simulink model "Copter_Plane_h2g_4_and_1_20210113"  (R2020b)
settings: Solver=ode1  StartTime=0.0  StopTime=50  FixedStep=dt  RelTol=1e-3
values from neighbouring files (symbols this model uses):
  HD = 180/pi    (= 57.2957795131)    [mode_data.m]
undefined symbols (not defined in the file or in its folder): center_WP, GRAVITY_MSS, gyro_x, gyro_y, gyro_z, J, k_aileron, k_aileronL, k_aileronR, k_elevator, k_flap, k_rudder, Kd, Ku, Ld, Ldx, Ldy, Lu, Lux, Luy, m_kg, Newton, pid_vel_xy_derivative, pid_vel_xy_input, pid_vel_xy_integrator, pitch, POSCONTROL_ACC_Z_D, POSCONTROL_ACC_Z_P, POSCONTROL_VEL_XY_D, POSCONTROL_VEL_XY_P, pwm_max, pwm_min, pwm_out, pwm_tail, Qd, QLd, QLdx, QLdy, QLu, QLux, QLuy, Qu, Raphson, roll, tail_tilt, vel_desired, yaw
libraries: shared6dofsys x3, sharedutil x1, simulink x1, aerolibasang x1
(part 3 of 3)

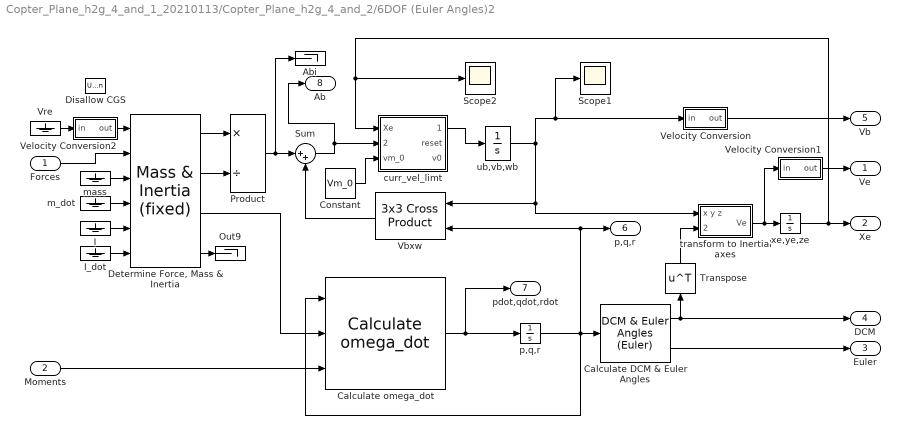
== system Copter_Plane_h2g_4_and_1_20210113/Copter_Plane_h2g_4_and_2/6DOF (Euler Angles)2 ==
  Forces : Inport  Unit=N  PortDimensions=3
  Moments : Inport  Port=2  Unit=N*m  PortDimensions=3
  Abi : Terminator
  Calculate DCM & Euler Angles : shared6dofsys/DCM & Euler Angles (Euler)  aMode=aMode
      settings: SourceProductBaseCode=AE,PW,MT,UV,VE,VP
  Calculate omega_dot : shared6dofsys/Calculate omega_dot  aMode=aMode
      settings: SourceProductBaseCode=AE,PW,MT,UV,VE,VP
  Constant : Constant  Value=Vm_0
  "Determine Force, Mass & Inertia" : shared6dofsys/Mass & Inertia (fixed)  aMode=aMode
      settings: SourceProductBaseCode=AE,PW,MT,UV,VE,VP
  Disallow CGS : UnitConfiguration  UnitSystemsStr=English,SI,SI (extended)  AllowAllUnitSystems=off
  I : Ground
  I_dot : Ground
  Out9 : Terminator
  Product : Product  Inputs=*/  SaturateOnIntegerOverflow=on  OutDataTypeStr=Inherit: Same as first input
  Scope1 : Scope
  Scope2 : Scope
  Sum : Sum  Inputs=|++  SaturateOnIntegerOverflow=on
  Transpose : Math  Operator=transpose  SignedPower=on  SaturateOnIntegerOverflow=on
  Vbxw : sharedutil/3x3 Cross Product  aMode=aMode
      settings: SourceProductBaseCode=AE,PW,MT,UV,VE,VP
  Velocity Conversion : Subsystem
  Velocity Conversion1 : Subsystem
  Velocity Conversion2 : Subsystem
  Vre : Ground
  curr_vel_limt : MATLAB Function  TreatAsAtomicUnit=on
  m_dot : Ground
  mass : Ground
  "p,q,r " : Integrator  InitialCondition=pm_0  ContinuousStateAttributes=pm_statename
  "transform to Inertial axes " : Subsystem  mask(Vector Transformation){}
      mask Display: disp('L_EB')
  ub,vb,wb : Integrator  InitialCondition=Vm_0  UpperSaturationLimit=[inf inf 0]  ContinuousStateAttributes=Vm_statename
  xe,ye,ze : Integrator  InitialCondition=xme_0  ContinuousStateAttributes=xme_statename
  Ve : Outport  Unit=m/s  VectorParamsAs1DForOutWhenUnconnected=off
  Xe : Outport  Port=2  Unit=m  VectorParamsAs1DForOutWhenUnconnected=off
  Euler : Outport  Port=3  Unit=rad  VectorParamsAs1DForOutWhenUnconnected=off
  DCM : Outport  Port=4  Unit=1  VectorParamsAs1DForOutWhenUnconnected=off
  Vb : Outport  Port=5  Unit=m/s  VectorParamsAs1DForOutWhenUnconnected=off
  p,q,r : Outport  Port=6  Unit=rad/s  VectorParamsAs1DForOutWhenUnconnected=off
  pdot,qdot,rdot : Outport  Port=7  Unit=rad/s^2  VectorParamsAs1DForOutWhenUnconnected=off
  Ab : Outport  Port=8  Unit=m/s^2  VectorParamsAs1DForOutWhenUnconnected=off
  wires:
  Velocity Conversion1/1(out) -> Ve/1
  Sum/1 -> Ab/1, curr_vel_limt/2(accel_in)
  ub,vb,wb/1 -> "transform to Inertial axes "/1(x y z), Vbxw/1, Scope1/1, Velocity Conversion/1(in)
  Velocity Conversion/1(out) -> Vb/1
  Velocity Conversion2/1(out) -> "Determine Force, Mass & Inertia"/1
  Vre/1 -> Velocity Conversion2/1(in)
  "Determine Force, Mass & Inertia"/1 -> Product/1
  I_dot/1 -> "Determine Force, Mass & Inertia"/6
  I/1 -> "Determine Force, Mass & Inertia"/5
  Calculate omega_dot/1 -> "p,q,r "/1, pdot,qdot,rdot/1
  "Determine Force, Mass & Inertia"/4 -> Out9/1
  m_dot/1 -> "Determine Force, Mass & Inertia"/4
  "Determine Force, Mass & Inertia"/2 -> Product/2
  mass/1 -> "Determine Force, Mass & Inertia"/3
  Transpose/1 -> "transform to Inertial axes "/2(transform coefficients)
  Calculate DCM & Euler Angles/1 -> Transpose/1, DCM/1
  Product/1 -> Sum/1, Abi/1
  Forces/1 -> "Determine Force, Mass & Inertia"/2
  Moments/1 -> Calculate omega_dot/3
  "p,q,r "/1 -> Calculate DCM & Euler Angles/1, Calculate omega_dot/1, p,q,r/1, Vbxw/2
  "transform to Inertial axes "/1(Ve) -> xe,ye,ze/1, Velocity Conversion1/1(in)
  xe,ye,ze/1 -> Scope2/1, curr_vel_limt/1(Xe), Xe/1
  Vbxw/1 -> Sum/2
  Calculate DCM & Euler Angles/2 -> Euler/1
  "Determine Force, Mass & Inertia"/3 -> Calculate omega_dot/2
  curr_vel_limt/1(accel_o) -> ub,vb,wb/1
  Constant/1 -> curr_vel_limt/3(vm_0)

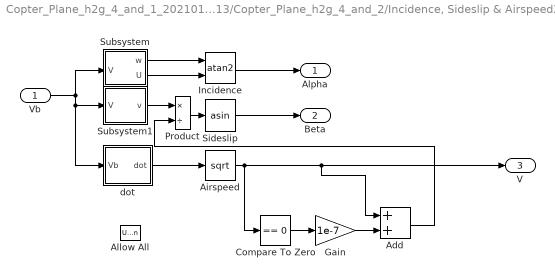
== system Copter_Plane_h2g_4_and_1_20210113/Copter_Plane_h2g_4_and_2/Incidence, Sideslip & Airspeed2 ==
  Vb : Inport
  Add : Sum
  Airspeed : Sqrt  AlgorithmType=Newton-Raphson  SaturateOnIntegerOverflow=on
  Allow All : UnitConfiguration  UnitSystemsStr=English,SI,SI (extended)  AllowAllUnitSystems=off
  Compare To Zero : simulink/Logic and Bit Operations/Compare To Zero  relop===  OutDataTypeStr=boolean
  Gain : Gain  Gain=1e-7
  Incidence : Trigonometry  Operator=atan2
  Product : Product  Inputs=*/  SaturateOnIntegerOverflow=on  OutDataTypeStr=Inherit: Same as first input
  Sideslip : Trigonometry  Operator=asin
  Subsystem : Subsystem
  Subsystem1 : Subsystem
  dot : Subsystem
  Alpha : Outport  Unit=rad  InitialOutput=0  VectorParamsAs1DForOutWhenUnconnected=off
  Beta : Outport  Port=2  Unit=rad  InitialOutput=0  VectorParamsAs1DForOutWhenUnconnected=off
  V : Outport  Port=3  InitialOutput=0  VectorParamsAs1DForOutWhenUnconnected=off
  wires:
  Product/1 -> Sideslip/1
  Subsystem/1(w) -> Incidence/1
  Subsystem/2(U) -> Incidence/2
  dot/1(dot) -> Airspeed/1
  Airspeed/1 -> Compare To Zero/1, Add/1, V/1
  Incidence/1 -> Alpha/1
  Vb/1 -> Subsystem/1(V), Subsystem1/1(V), dot/1(Vb)
  Sideslip/1 -> Beta/1
  Subsystem1/1(v) -> Product/1
  Compare To Zero/1 -> Gain/1
  Gain/1 -> Add/2
  Add/1 -> Product/2

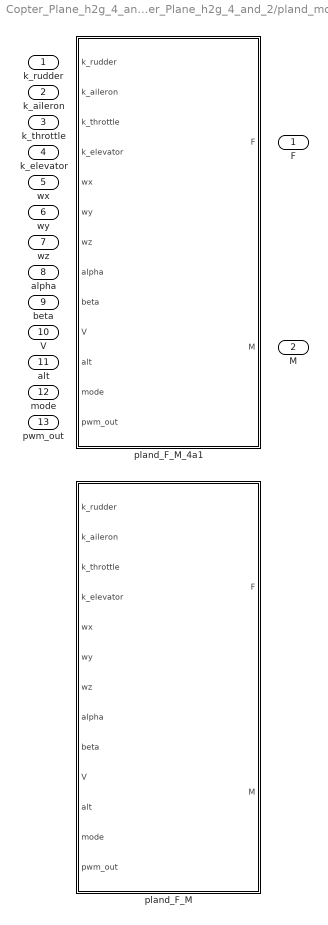
== system Copter_Plane_h2g_4_and_1_20210113/Copter_Plane_h2g_4_and_2/pland_mode ==
  k_rudder : Inport
  k_aileron : Inport  Port=2
  k_throttle : Inport  Port=3
  k_elevator : Inport  Port=4
  wx : Inport  Port=5
  wy : Inport  Port=6
  wz : Inport  Port=7
  alpha : Inport  Port=8
  beta : Inport  Port=9
  V : Inport  Port=10
  alt : Inport  Port=11
  mode : Inport  Port=12
  pwm_out : Inport  Port=13
  pland_F_M : MATLAB Function  TreatAsAtomicUnit=on  VariantControl=plane_mode==ENUM_plane_mode.V1000
  pland_F_M_4a1 : MATLAB Function  TreatAsAtomicUnit=on  VariantControl=plane_mode==ENUM_plane_mode.V10||plane_mode==ENUM_plane_mode.V10s
  F : Outport
  M : Outport  Port=2

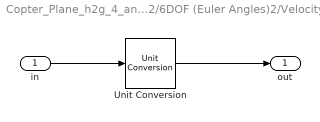
== system Copter_Plane_h2g_4_and_1_20210113/Copter_Plane_h2g_4_and_2/6DOF (Euler Angles)2/Velocity Conversion ==
  in : Inport  Unit=m/s
  Unit Conversion : UnitConversion
  out : Outport  VectorParamsAs1DForOutWhenUnconnected=off
  wires:
  Unit Conversion/1 -> out/1
  in/1 -> Unit Conversion/1

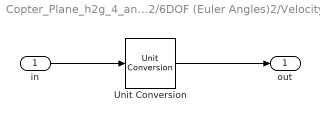
== system Copter_Plane_h2g_4_and_1_20210113/Copter_Plane_h2g_4_and_2/6DOF (Euler Angles)2/Velocity Conversion1 ==
  in : Inport  Unit=m/s
  Unit Conversion : UnitConversion
  out : Outport  VectorParamsAs1DForOutWhenUnconnected=off
  wires:
  Unit Conversion/1 -> out/1
  in/1 -> Unit Conversion/1

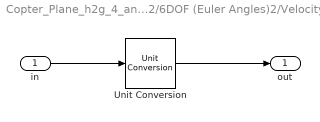
== system Copter_Plane_h2g_4_and_1_20210113/Copter_Plane_h2g_4_and_2/6DOF (Euler Angles)2/Velocity Conversion2 ==
  in : Inport  Unit=m/s
  Unit Conversion : UnitConversion
  out : Outport  Unit=m/s  VectorParamsAs1DForOutWhenUnconnected=off
  wires:
  Unit Conversion/1 -> out/1
  in/1 -> Unit Conversion/1

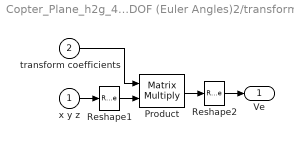
== system Copter_Plane_h2g_4_and_1_20210113/Copter_Plane_h2g_4_and_2/6DOF (Euler Angles)2/transform to Inertial axes  ==
  x y z : Inport
  transform coefficients : Inport  Port=2
  Product : Product  Multiplication=Matrix(*)  InputSameDT=on  SaturateOnIntegerOverflow=on  OutDataTypeStr=Inherit: Same as first input
  Reshape1 : Reshape  OutputDimensionality=Column vector (2-D)
  Reshape2 : Reshape
  Ve : Outport  VectorParamsAs1DForOutWhenUnconnected=off
  wires:
  Reshape2/1 -> Ve/1
  Reshape1/1 -> Product/2
  x y z/1 -> Reshape1/1
  transform coefficients/1 -> Product/1
  Product/1 -> Reshape2/1

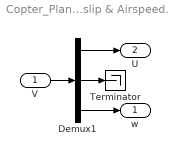
== system Copter_Plane_h2g_4_and_1_20210113/Copter_Plane_h2g_4_and_2/Incidence, Sideslip & Airspeed2/Subsystem ==
  V : Inport
  Demux1 : Demux  Outputs=3
      settings: DisplayOption=none
  Terminator : Terminator
  w : Outport  VectorParamsAs1DForOutWhenUnconnected=off
  U : Outport  Port=2  VectorParamsAs1DForOutWhenUnconnected=off
  wires:
  Demux1/3 -> w/1
  Demux1/2 -> Terminator/1
  V/1 -> Demux1/1
  Demux1/1 -> U/1

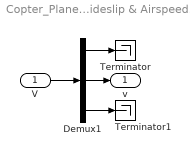
== system Copter_Plane_h2g_4_and_1_20210113/Copter_Plane_h2g_4_and_2/Incidence, Sideslip & Airspeed2/Subsystem1 ==
  V : Inport
  Demux1 : Demux  Outputs=3
      settings: DisplayOption=none
  Terminator : Terminator
  Terminator1 : Terminator
  v : Outport  VectorParamsAs1DForOutWhenUnconnected=off
  wires:
  Demux1/1 -> Terminator/1
  Demux1/3 -> Terminator1/1
  V/1 -> Demux1/1
  Demux1/2 -> v/1

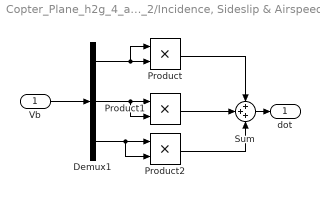
== system Copter_Plane_h2g_4_and_1_20210113/Copter_Plane_h2g_4_and_2/Incidence, Sideslip & Airspeed2/dot ==
  Vb : Inport
  Demux1 : Demux  Outputs=3
  Product : Product  RndMeth=Zero
  Product1 : Product  RndMeth=Zero
  Product2 : Product  RndMeth=Zero
  Sum : Sum  Inputs=+++
  dot : Outport  VectorParamsAs1DForOutWhenUnconnected=off
  wires:
  Product2/1 -> Sum/3
  Demux1/3 -> Product2/2, Product2/1
  Product/1 -> Sum/1
  Product1/1 -> Sum/2
  Sum/1 -> dot/1
  Vb/1 -> Demux1/1
  Demux1/1 -> Product/2, Product/1
  Demux1/2 -> Product1/1, Product1/2

== matlab function Copter_Plane_h2g_4_and_1_20210113/Copter_Plane_h2g_4_and_2/pland_mode/pland_F_M_4a1 ==
  settings: updateMethod=DISCRETE
  data: F output; k_rudder input; k_aileron input; k_throttle input; k_elevator input; wx input; wy input; wz input; alpha input; beta input; V input; alt input; M output; mode input; pwm_out input; Ku parameter; Kd parameter; Lux parameter; Luy parameter; Ldx parameter; Ldy parameter; Lu parameter; Ld parameter; pwm_min parameter; pwm_max parameter; Qu parameter; Qd parameter; tail_tilt data_store_memory; QLux parameter; QLuy parameter; QLu parameter; QLdx parameter; QLdy parameter; QLd parameter; pwm_tail data_store_memory
function [F,M]   = pland_F_M_4a1(k_rudder,k_aileron,k_throttle,k_elevator,wx,wy,wz,alpha,beta,V,alt,mode,pwm_out, Ku, Kd, Lux, Luy, Ldx, Ldy, Lu, Ld, pwm_min, pwm_max, Qu, Qd, QLux, QLuy, QLu, QLdx, QLdy, QLd)
    
%鎺ㄥ姏妯″瀷锛孴hr=throttle_dem*Tmax锛宼hrottle_dem=24N銆俓n%闃诲姏妯″瀷锛孋x_Sref=Cx_Sref_alpha*alpha,Cx_Sref_alpha=0.007;
%鍗囧姏妯″瀷  Cy_Sref=Cy_Sref_alpha*(alpha0+alpha),Cy_Sref_alpha=0.022,alpha0=5;
%%%%%%%%%%%%%%%%%%%%%%%%%%%%%%%%%%%%%%%%%%%%%%%%%%%%%%%%%%%%%%%%%%%%%%%
global tail_tilt
global pwm_tail
Tmax=26*9.8*0.6;
HD=180/pi;
% if(abs(alpha)>20/HD||V<8)
%     V=0;
% end
if(V<8)
    V=0;
end

alpha=constrain_value(alpha,-10/HD,10/HD);
beta=constrain_value(beta,-10/HD,10/HD);
Cx_Sref_alpha=-1.274/2/10;%8/144.5
Cz_Sref_alpha=-1.274/2;
Cy_Sref_beta=-1.274/2/10;
alpha0=2/HD;
Cx_Sref=Cx_Sref_alpha*20;
Cy_Sref=Cy_Sref_beta*(beta)*HD;
Cz_Sref=Cz_Sref_alpha*(alpha+alpha0)*HD;

Sbw=[cos(alpha)*cos(beta)   -cos(alpha)*sin(beta)   -sin(alpha)
    sin(beta)               cos(beta)               0
    sin(alpha)*cos(beta)    -sin(alpha)*sin(beta)   cos(alpha)];
[~,~,rho,~] = atom_mode(alt+2000);
q=0.5*rho*V*V;
D=q*Cx_Sref;%+k_throttle*Tmax;
C=q*Cy_Sref;
L=q*Cz_Sref;
Fw=[D; C; L];
Fb=Sbw*Fw;
TF=(pwm_tail-pwm_min)/(pwm_max-pwm_min)*Tmax;
F_Plane=Fb+[TF;0;0];
% F_Plane=Fb;

%%%%%%%%%%%%%%%%%%%%%%%%%%%%%%%%%%%%%%%%%%%%%%%%%
dl=0.1;
Mby=Fb(3)*dl;
Mbz=-Fb(2)*dl;
%%%%%%%%%%%%%%%%%%%%%%%%%
dmxa=71.8362;    %(2*pi*5)^2*Jx/HD
dmx_wx=0.1;
%%%%%%%%%%%%%%%%%%%%%%%%%%%
dmya=q*Cz_Sref_alpha*dl;  %(2*pi*1.5)^2*Jy/HD
dmye=-dmya/2;
dmy_wy=0.2;
%%%%%%%%%%%%%%%%%%%%%%%%%
dmzb=-q*Cy_Sref_beta*dl;    %(2*pi*5)^2*Jx/HD
dmzr=dmzb*0.3;
dmz_wz=0.2;
%%%%%%%%%%%%%%%%%%%%%%%%
Mx=dmxa*k_aileron/100          -dmx_wx*wx;
My=dmye*(k_elevator+680)/100  +Mby   -dmy_wy*wy;
% My=dmye*(k_elevator)/100  +Mby   -dmy_wy*wy;
Mz=dmzr*k_rudder/100    +Mbz   -dmz_wz*wz;
M_Plane=[Mx; My ;Mz];
%%%%%%%%%%%%%%%%%%%%%%%%%%%%%%%%%%%%%%%%%%%%%%%%%%%%%%%%%%%%%%%%%%%
%%%%%%%%%%%%%%%%%%%%%%%%%%%%%%%%%%%%%%%%%%%%%%%%%%%%%%%%%%%%%%%%%%%%%
%%%%%%%%%%%%%%%%%%%%%%%%%%%%%%%%%%%%%%%%%%%%%%%%%%%%%%%%%%%%%%%%%%%%%
Ku_v10=26*9.8*3/4;
F1=(pwm_out(1)-pwm_min)/(pwm_max-pwm_min)*Ku_v10;
F2=(pwm_out(2)-pwm_min)/(pwm_max-pwm_min)*Ku_v10;
F3=(pwm_out(3)-pwm_min)/(pwm_max-pwm_min)*Ku_v10;
F4=(pwm_out(4)-pwm_min)/(pwm_max-pwm_min)*Ku_v10;

tail_tilt_temp=constrain_value(tail_tilt,-9000,700);

F24x_g=(F2+F4)*sind(-tail_tilt_temp/100);
F24z_g=(F2+F4)*cosd(-tail_tilt_temp/100);

F_copter=[F24x_g; 0 ;-(F1+F3+F24z_g)];
L_v10=0.5;
Q=4.5;
Mx=(-F1+F3)*L_v10+(F2-F4)*L_v10;
% My=(F1+F3)*Luy+(-F2-F4)*Ldy;
My=(F1+F3)*L_v10+(-F2-F4)*L_v10*cosd(-tail_tilt_temp/100);
Mz=(-F1+F3)*L_v10*sind(Q)+(-F2+F4)*L_v10*sind(Q);%0.1736=sind(10)  0.1071= Ld*900*sind(10)/(Lu*1600)
Mz_g=(F2-F4)*Ldx*sind(-tail_tilt_temp/100);
% Mz_g=0;
Mz=Mz+Mz_g;
M_copter=[Mx; My; Mz];
%%%%%%%%%%%%%%%%%%%%%%%%%%%%%%%%%%%%%%%%%%%%%%%%%%%%%%%
%% 0 :copter Stabilize,1:copter althold ,2:copter poshold,3:Plane Stabilize 4:Plane TECS; 5：Plane L1
    F=F_copter+F_Plane;
    M=M_copter+M_Plane;
    
%     F=F_copter;
%     M=M_copter;
%%%%%%%%%%%%%%%%%%%%%%%%%%%%%%%%%%%%%%%%%%%%%%%%%%%%%%%%%%%%
end

== matlab function Copter_Plane_h2g_4_and_1_20210113/Copter_Plane_h2g_4_and_2/pland_mode/pland_F_M ==
  settings: updateMethod=DISCRETE
  data: F output; k_rudder input; k_aileron input; k_throttle input; k_elevator input; wx input; wy input; wz input; alpha input; beta input; V input; alt input; M output; mode input; pwm_out input; Ku parameter; Kd parameter; Lux parameter; Luy parameter; Ldx parameter; Ldy parameter; Lu parameter; Ld parameter; pwm_min parameter; pwm_max parameter; Qu parameter; Qd parameter; tail_tilt data_store_memory; QLux parameter; QLuy parameter; QLu parameter; QLdx parameter; QLdy parameter; QLd parameter; pwm_tail data_store_memory
function [F,M]   = pland_F_M(k_rudder,k_aileron,k_throttle,k_elevator,wx,wy,wz,alpha,beta,V,alt,mode,pwm_out, Ku, Kd, Lux, Luy, Ldx, Ldy, Lu, Ld, pwm_min, pwm_max, Qu, Qd, QLux, QLuy, QLu, QLdx, QLdy, QLd)
    
%鎺ㄥ姏妯″瀷锛孴hr=throttle_dem*Tmax锛宼hrottle_dem=24N銆俓n%闃诲姏妯″瀷锛孋x_Sref=Cx_Sref_alpha*alpha,Cx_Sref_alpha=0.007;
%鍗囧姏妯″瀷  Cy_Sref=Cy_Sref_alpha*(alpha0+alpha),Cy_Sref_alpha=0.022,alpha0=5;
%%%%%%%%%%%%%%%%%%%%%%%%%%%%%%%%%%%%%%%%%%%%%%%%%%%%%%%%%%%%%%%%%%%%%%%
global tail_tilt
Tmax=36;
HD=180/pi;
% if(abs(alpha)>20/HD||V<8)
%     V=0;
% end
if(V<8)
    V=0;
end

alpha=constrain_value(alpha,-10/HD,10/HD);
beta=constrain_value(beta,-10/HD,10/HD);
Cx_Sref_alpha=-0.0554;%8/144.5
Cz_Sref_alpha=-0.1075*0.86;
Cy_Sref_beta=-0.1075*0.86*0.1;
alpha0=2/HD;
Cx_Sref=Cx_Sref_alpha;
Cy_Sref=Cy_Sref_beta*(beta)*HD;
Cz_Sref=Cz_Sref_alpha*(alpha+alpha0)*HD;

Sbw=[cos(alpha)*cos(beta)   -cos(alpha)*sin(beta)   -sin(alpha)
    sin(beta)               cos(beta)               0
    sin(alpha)*cos(beta)    -sin(alpha)*sin(beta)   cos(alpha)];
[~,~,rho,~] = atom_mode(alt+2000);
q=0.5*rho*V*V;
D=q*Cx_Sref;%+k_throttle*Tmax;
C=q*Cy_Sref;
L=q*Cz_Sref;
Fw=[D; C; L];
Fb=Sbw*Fw;
% F_Plane=Fb+[k_throttle*Tmax;0;0];
F_Plane=Fb;

%%%%%%%%%%%%%%%%%%%%%%%%%%%%%%%%%%%%%%%%%%%%%%%%%
dl=0.1;
Mby=Fb(3)*dl;
Mbz=-Fb(2)*dl;
%%%%%%%%%%%%%%%%%%%%%%%%%
dmxa=3.2078;    %(2*pi*5)^2*Jx/HD
dmx_wx=0.1;
%%%%%%%%%%%%%%%%%%%%%%%%%%%
dmya=q*Cz_Sref_alpha*dl;  %(2*pi*1.5)^2*Jy/HD
dmye=-dmya/2;
dmy_wy=0.2;
%%%%%%%%%%%%%%%%%%%%%%%%%
dmzb=-q*Cy_Sref_beta*dl;    %(2*pi*5)^2*Jx/HD
dmzr=dmzb*0.3;
dmz_wz=0.2;
%%%%%%%%%%%%%%%%%%%%%%%%
Mx=dmxa*k_aileron/100          -dmx_wx*wx;
My=dmye*(k_elevator+680)/100  +Mby   -dmy_wy*wy;
% My=dmye*(k_elevator)/100  +Mby   -dmy_wy*wy;
Mz=dmzr*k_rudder/100    +Mbz   -dmz_wz*wz;
M_Plane=[Mx; My ;Mz];
%%%%%%%%%%%%%%%%%%%%%%%%%%%%%%%%%%%%%%%%%%%%%%%%%%%%%%%%%%%%%%%%%%%
%%%%%%%%%%%%%%%%%%%%%%%%%%%%%%%%%%%%%%%%%%%%%%%%%%%%%%%%%%%%%%%%%%%%%
%%%%%%%%%%%%%%%%%%%%%%%%%%%%%%%%%%%%%%%%%%%%%%%%%%%%%%%%%%%%%%%%%%%%%
% Kd=Kd;
F1=(pwm_out(1)-pwm_min)/(pwm_max-pwm_min)*Ku;
F2=(pwm_out(2)-pwm_min)/(pwm_max-pwm_min)*Kd;
F3=(pwm_out(3)-pwm_min)/(pwm_max-pwm_min)*Ku;
F4=(pwm_out(4)-pwm_min)/(pwm_max-pwm_min)*Kd;
%  F2=0;
tail_tilt_temp=constrain_value(tail_tilt,-9000,700);

F24x_g=(F2+F4)*sind(-tail_tilt_temp/100);
F24z_g=(F2+F4)*cosd(-tail_tilt_temp/100);

F_copter=[F24x_g; 0 ;-(F1+F3+F24z_g)];
Mx=(-F1+F3)*Lux+(F2-F4)*Ldx;
% My=(F1+F3)*Luy+(-F2-F4)*Ldy;
My=(F1+F3)*Luy+(-F2-F4)*Ldy*cosd(-tail_tilt_temp/100);
Mz=(-F1+F3)*Lu*sind(Qu)+(-F2+F4)*Ld*sind(Qd);%0.1736=sind(10)  0.1071= Ld*900*sind(10)/(Lu*1600)
Mz_g=(F2-F4)*Ldx*sind(-tail_tilt_temp/100);
% Mz_g=0;
Mz=Mz+Mz_g;
M_copter=[Mx; My; Mz];
%%%%%%%%%%%%%%%%%%%%%%%%%%%%%%%%%%%%%%%%%%%%%%%%%%%%%%%
%% 0 :copter Stabilize,1:copter althold ,2:copter poshold,3:Plane Stabilize 4:Plane TECS; 5：Plane L1
    F=F_copter+F_Plane;
    M=M_copter+M_Plane;
    
%     F=F_copter;
%     M=M_copter;
%%%%%%%%%%%%%%%%%%%%%%%%%%%%%%%%%%%%%%%%%%%%%%%%%%%%%%%%%%%%
end

== matlab function Copter_Plane_h2g_4_and_1_20210113/Copter_Plane_h2g_4_and_2/6DOF (Euler Angles)2/curr_vel_limt ==
  data: Xe input; accel_in input; accel_o output; reset output; vm_0 input; v0 output
function [accel_o,reset,v0] = accel_limt(Xe,accel_in,vm_0)

if((Xe(3)>0))
    accel_o=[accel_in(1) accel_in(2)  0]';
    v0=[0 0 0]';
    reset=1;
else
    accel_o=accel_in;
    reset=0;
    v0=vm_0;
end

== matlab function Copter_Plane_h2g_4_and_1_20210113/Copter_Plane_h2g_4_and_2/MATLAB Function ==
  data: PWM input; PWM_n output
function PWM_n      = fcn(PWM)

PWM_n=(PWM-1000)/1000;

== matlab function Copter_Plane_h2g_4_and_1_20210113/Copter_Plane_h2g_4_and_2/pland_F_M ==
  settings: updateMethod=DISCRETE
  data: F output; k_rudder input; k_aileron input; k_throttle input; k_elevator input; wx input; wy input; wz input; alpha input; beta input; V input; alt input; M output; mode input; pwm_out input; Ku parameter; Kd parameter; Lux parameter; Luy parameter; Ldx parameter; Ldy parameter; Lu parameter; Ld parameter; pwm_min parameter; pwm_max parameter; Qu parameter; Qd parameter; tail_tilt data_store_memory; QLux parameter; QLuy parameter; QLu parameter; QLdx parameter; QLdy parameter; QLd parameter; pwm_tail data_store_memory; F_copter output; F_Plane output; M_copter output; M_Plane output
function [F,M,F_copter,F_Plane,M_copter,M_Plane]   = pland_F_M(k_rudder,k_aileron,k_throttle,k_elevator,wx,wy,wz,alpha,beta,V,alt,mode,pwm_out, Ku, Kd, Lux, Luy, Ldx, Ldy, Lu, Ld, pwm_min, pwm_max, Qu, Qd, QLux, QLuy, QLu, QLdx, QLdy, QLd)
    
%鎺ㄥ姏妯″瀷锛孴hr=throttle_dem*Tmax锛宼hrottle_dem=24N銆俓n%闃诲姏妯″瀷锛孋x_Sref=Cx_Sref_alpha*alpha,Cx_Sref_alpha=0.007;
%鍗囧姏妯″瀷  Cy_Sref=Cy_Sref_alpha*(alpha0+alpha),Cy_Sref_alpha=0.022,alpha0=5;
%%%%%%%%%%%%%%%%%%%%%%%%%%%%%%%%%%%%%%%%%%%%%%%%%%%%%%%%%%%%%%%%%%%%%%%
global tail_tilt
Tmax=36;
HD=180/pi;
% if(abs(alpha)>20/HD||V<8)
%     V=0;
% end
if(V<8)
    V=0;
end

alpha=constrain_value(alpha,-10/HD,10/HD);
beta=constrain_value(beta,-10/HD,10/HD);
Cx_Sref_alpha=-0.0554;%8/144.5
Cz_Sref_alpha=-0.1075*0.86;
Cy_Sref_beta=-0.1075*0.86*0.1;
alpha0=2/HD;
Cx_Sref=Cx_Sref_alpha;
Cy_Sref=Cy_Sref_beta*(beta)*HD;
Cz_Sref=Cz_Sref_alpha*(alpha+alpha0)*HD;

Sbw=[cos(alpha)*cos(beta)   -cos(alpha)*sin(beta)   -sin(alpha)
    sin(beta)               cos(beta)               0
    sin(alpha)*cos(beta)    -sin(alpha)*sin(beta)   cos(alpha)];
[~,~,rho,~] = atom_mode(alt+2000);
q=0.5*rho*V*V;
D=q*Cx_Sref;%+k_throttle*Tmax;
C=q*Cy_Sref;
L=q*Cz_Sref;
Fw=[D; C; L];
Fb=Sbw*Fw;
% F_Plane=Fb+[k_throttle*Tmax;0;0];
F_Plane=Fb ;

%%%%%%%%%%%%%%%%%%%%%%%%%%%%%%%%%%%%%%%%%%%%%%%%%
dl=0.1;
Mby=Fb(3)*dl;
Mbz=-Fb(2)*dl;
%%%%%%%%%%%%%%%%%%%%%%%%%
dmxa=3.2078;    %(2*pi*5)^2*Jx/HD
dmx_wx=0.1;
%%%%%%%%%%%%%%%%%%%%%%%%%%%
dmya=q*Cz_Sref_alpha*dl;  %(2*pi*1.5)^2*Jy/HD
dmye=-dmya/2;
dmy_wy=0.2;
%%%%%%%%%%%%%%%%%%%%%%%%%
dmzb=-q*Cy_Sref_beta*dl;    %(2*pi*5)^2*Jx/HD
dmzr=dmzb*0.3;
dmz_wz=0.2;
%%%%%%%%%%%%%%%%%%%%%%%%
Mx=dmxa*k_aileron/100          -dmx_wx*wx;
My=dmye*(k_elevator+680)/100  +Mby   -dmy_wy*wy;
% My=dmye*(k_elevator)/100  +Mby   -dmy_wy*wy;
Mz=dmzr*k_rudder/100    +Mbz   -dmz_wz*wz;
M_Plane=[Mx; My ;Mz];
%%%%%%%%%%%%%%%%%%%%%%%%%%%%%%%%%%%%%%%%%%%%%%%%%%%%%%%%%%%%%%%%%%%
%%%%%%%%%%%%%%%%%%%%%%%%%%%%%%%%%%%%%%%%%%%%%%%%%%%%%%%%%%%%%%%%%%%%%
%%%%%%%%%%%%%%%%%%%%%%%%%%%%%%%%%%%%%%%%%%%%%%%%%%%%%%%%%%%%%%%%%%%%%
% Kd=Kd;
F1=(pwm_out(1)-pwm_min)/(pwm_max-pwm_min)*Ku;
F2=(pwm_out(2)-pwm_min)/(pwm_max-pwm_min)*Kd;
F3=(pwm_out(3)-pwm_min)/(pwm_max-pwm_min)*Ku;
F4=(pwm_out(4)-pwm_min)/(pwm_max-pwm_min)*Kd;
%  F2=0;
tail_tilt_temp=constrain_value(tail_tilt,-9000,700);

F24x_g=(F2+F4)*sind(-tail_tilt_temp/100);
F24z_g=(F2+F4)*cosd(-tail_tilt_temp/100);

F_copter=[F24x_g; 0 ;-(F1+F3+F24z_g)];
Mx=(-F1+F3)*Lux+(F2-F4)*Ldx;
% My=(F1+F3)*Luy+(-F2-F4)*Ldy;
My=(F1+F3)*Luy+(-F2-F4)*Ldy*cosd(-tail_tilt_temp/100);
Mz=(-F1+F3)*Lu*sind(Qu)+(-F2+F4)*Ld*sind(Qd);%0.1736=sind(10)  0.1071= Ld*900*sind(10)/(Lu*1600)
Mz_g=(F2-F4)*Ldx*sind(-tail_tilt_temp/100);
% Mz_g=0;
Mz=Mz+Mz_g;
M_copter=[Mx; My; Mz];
%%%%%%%%%%%%%%%%%%%%%%%%%%%%%%%%%%%%%%%%%%%%%%%%%%%%%%%
%% 0 :copter Stabilize,1:copter althold ,2:copter poshold,3:Plane Stabilize 4:Plane TECS; 5：Plane L1
    F=F_copter+F_Plane;
    M=M_copter+M_Plane;
    
%     F=F_copter;
%     M=M_copter;
%%%%%%%%%%%%%%%%%%%%%%%%%%%%%%%%%%%%%%%%%%%%%%%%%%%%%%%%%%%%
end

== matlab function Copter_Plane_h2g_4_and_1_20210113/Copter_Plane_h2g_4_and_2/Location_offset1 ==
  data: center_WP input; current_loc output; ofs_north input; ofs_east input; LOCATION_SCALING_FACTOR_INV data_store_memory; HD data_store_memory
function current_loc=Location_offset( center_WP,ofs_north,  ofs_east)

current_loc=Location_offset( center_WP,ofs_north,  ofs_east);

== matlab function Copter_Plane_h2g_4_and_1_20210113/Copter_Plane_h2g_4_and_2/get_vector_xy_from_origin_NE1 ==
  data: loc input; vec_ne output; loc_origin input; LOCATION_SCALING_FACTOR_INV data_store_memory; HD data_store_memory; LOCATION_SCALING_FACTOR data_store_memory
function vec_ne=get_vector_xy_from_origin_NE( loc,loc_origin) 

vec_ne=get_vector_xy_from_origin_NE( loc,loc_origin ) ;

== matlab function Copter_Plane_h2g_4_and_1_20210113/Copter_Plane_h2g_4_and_2/input_euler_angle_roll_pitch_euler_rate_yaw4 ==
  data: gains_I_pitch data_store_memory; gains_tau_pitch data_store_memory; gains_P_pitch data_store_memory; gains_D_pitch data_store_memory; gains_imax_pitch data_store_memory; gains_FF_pitch data_store_memory; airspeed_min data_store_memory; last_out_pitch data_store_memory; pid_info_I_pitch data_store_memory; pid_info_P_pitch data_store_memory; pid_info_FF_pitch data_store_memory; pid_info_D_pitch data_store_memory; pid_info_desired_pitch data_store_memory; pid_info_actual_pitch data_store_memory; roll data_store_memory; pitch data_store_memory; roll_limit_cd data_store_memory; aspeed data_store_memory; max_rate_neg data_store_memory; gains_rmax_pitch data_store_memory; GRAVITY_MSS data_store_memory; roll_ff_pitch data_store_memory; HD data_store_memory; gains_D_roll data_store_memory; gains_FF_roll data_store_memory; gains_I_roll data_store_memory; gains_imax_roll data_store_memory; gains_P_roll data_store_memory; gains_rmax_roll data_store_memory; gains_tau_roll data_store_memory; last_out_roll data_store_memory; pid_info_actual_roll data_store_memory; pid_info_D_roll data_store_memory; pid_info_desired_roll data_store_memory; pid_info_FF_roll data_store_memory; pid_info_I_roll data_store_memory; pid_info_P_roll data_store_memory; accel_y data_store_memory; imax_yaw data_store_memory; integrator_yaw data_store_memory; K_A_yaw data_store_memory; K_D_last_yaw data_store_memory; K_D_yaw data_store_memory; K_FF_yaw data_store_memory; K_I_yaw data_store_memory; last_out_yaw data_store_memory; last_rate_hp_in_yaw data_store_memory; last_rate_hp_out_yaw data_store_memory; pid_info_D_yaw data_store_memory; pid_info_I_yaw data_store_memory; throttle_dem data_store_memory; pitch_dem data_store_memory; pitch_limit_min_cd data_store_memory; pitch_limit_max_cd data_store_memory; nav_pitch_cd data_store_memory; nav_roll_cd data_store_memory; inverted_flight data_store_memory; k_rudder data_store_memory; k_aileron data_store_memory; k_throttle data_store_memory; k_elevator data_store_memory; kff_throttle_to_pitch data_store_memory; highest_airspeed data_store_memory; scaling_speed data_store_memory; airspeed_max data_store_memory; latAccDem data_store_memory; smoothed_airspeed data_store_memory; aerodynamic_load_factor data_store_memory; kff_rudder_mix data_store_memory; TASmax data_store_memory; SKE_dem data_store_memory; TASmin data_store_memory; SPE_dem data_store_memory; SPE_est data_store_memory; SKE_est data_store_memory; STE_error data_store_memory; SPEdot_dem data_store_memory; SKEdot_dem data_store_memory; STEdot_min data_store_memory; STEdot_max data_store_memory; SPEdot data_store_memory; SKEdot data_store_memory; STEdotErrLast data_store_memory; timeConstant data_store_memory; throttle_cruise data_store_memory; rot_body_to_ned data_store_memory; rollComp data_store_memory; THRmaxf data_store_memory; THRminf data_store_memory; thrDamp data_store_memory; throttle_slewrate data_store_memory; last_throttle_dem data_store_memory; integGain data_store_memory; integTHR_state data_store_memory; maxClimbRate data_store_memory; minSinkRate data_store_memory; EAS_dem data_store_memory; hgt_dem data_store_memory; throttle_max data_store_memory; throttle_min data_store_memory; pitch_max data_store_memory; PITCHmaxf data_store_memory; pitch_min data_store_memory; PITCHminf data_store_memory; pitch_max_limit data_store_memory; TAS_dem data_store_memory; EAS2TAS data_store_memory; TAS_state data_store_memory; integDTAS_state data_store_memory; spdCompFiltOmega data_store_memory; vel_dot data_store_memory; TAS_dem_adj data_store_memory; TAS_rate_dem data_store_memory; hgt_dem_in_old data_store_memory; maxSinkRate data_store_memory; hgt_dem_prev data_store_memory; hgt_dem_adj_last data_store_memory; hgt_dem_adj data_store_memory; hgt_rate_dem data_store_memory; height data_store_memory; climb_rate data_store_memory; spdWeight data_store_memory; ptchDamp data_store_memory; pitch_dem_unc data_store_memory; integSEB_state data_store_memory; vertAccLim data_store_memory; last_pitch_dem data_store_memory; L1_damping data_store_memory; L1_period data_store_memory; current_loc data_store_memory; groundspeed_vector data_store_memory; target_bearing_cd data_store_memory; L1_dist data_store_memory; crosstrack_error data_store_memory; nav_bearing data_store_memory; L1_xtrack_i_gain data_store_memory; L1_xtrack_i_gain_prev data_store_memory; L1_xtrack_i data_store_memory; last_Nu data_store_memory; WPcircle data_store_memory; data_is_stale data_store_memory; bearing_error data_store_memory; LOCATION_SCALING_FACTOR data_store_memory; yaw data_store_memory; reverse data_store_memory; loiter_bank_limit data_store_memory; dt data_store_memory; roll_limit_cd_inint data_store_memory; accel_x data_store_memory; accel_z data_store_memory; Vz data_store_memory; vdot_filter data_store_memory; pwm_min data_store_memory; pwm_max data_store_memory; pwm_out data_store_memory; LOCATION_SCALING_FACTOR_INV data_store_memory; recalc_leash_z data_store_memory; leash_up_z data_store_memory; POSCONTROL_SPEED_UP data_store_memory; POSCONTROL_ACCEL_Z data_store_memory; POSCONTROL_POS_Z_P data_store_memory; leash_down_z data_store_memory; POSCONTROL_SPEED_DOWN data_store_memory; POSCONTROL_ACCELERATION_MIN data_store_memory; POSCONTROL_LEASH_LENGTH_MIN data_store_memory; limit_pos_up data_store_memory; limit_pos_down data_store_memory; pos_error data_store_memory; pos_target data_store_memory; curr_alt data_store_memory; vel_target data_store_memory; limit_vel_up data_store_memory; limit_vel_down data_store_memory; use_desvel_ff_z data_store_memory; reset_rate_to_accel_z data_store_memory; vel_desired data_store_memory; accel_desired data_store_memory; POSCONTROL_VEL_ERROR_CUTOFF_FREQ data_store_memory; vel_last data_store_memory; freeze_ff_z data_store_memory; vel_error data_store_memory; vel_error_input data_store_memory; curr_vel data_store_memory; accel_target data_store_memory; POSCONTROL_VEL_Z_P data_store_memory; reset_accel_to_throttle data_store_memory; accel_error data_store_memory; z_accel_meas data_store_memory; pid_accel_z_reset_filter data_store_memory; POSCONTROL_ACC_Z_FILT_HZ data_store_memory; pid_accel_z_input data_store_memory; pid_accel_z_derivative data_store_memory; POSCONTROL_ACC_Z_P data_store_memory; pid_accel_z_integrator data_store_memory; POSCONTROL_ACC_Z_IMAX data_store_memory; throttle_hover data_store_memory; throttle_lower data_store_memory; throttle_upper data_store_memory; POSCONTROL_ACC_Z_D data_store_memory; POSCONTROL_ACC_Z_I data_store_memory; throttle_thrust_max data_store_memory; althold_lean_angle_max data_store_memory; angle_limit_tc data_store_memory; angle_boost_enabled data_store_memory; angle_boost data_store_memory; throttle_rpy_mix data_store_memory; throttle_avg_max data_store_memory; AC_ATTITUDE_CONTROL_ANGLE_LIMIT_THROTTLE_MAX data_store_memory; POSCONTROL_POS_XY_P data_store_memory; curr_pos data_store_memory; leash data_store_memory; POSCONTROL_ACCEL_XY data_store_memory; POSCONTROL_VEL_XY_FILT_HZ data_store_memory; POSCONTROL_VEL_XY_FILT_D_HZ data_store_memory; pid_vel_xy_reset_filter data_store_memory; pid_vel_xy_input data_store_memory; pid_vel_xy_derivative data_store_memory; pid_vel_xy_integrator data_store_memory; POSCONTROL_VEL_XY_P data_store_memory; limit_accel_xy data_store_memory; motors_limit_throttle_upper data_store_memory; POSCONTROL_VEL_XY_I data_store_memory; POSCONTROL_VEL_XY_IMAX data_store_memory; POSCONTROL_VEL_XY_D data_store_memory; reset_accel_to_lean_xy data_store_memory; POSCONTROL_ACCEL_FILTER_HZ data_store_memory; accel_xy_input data_store_memory; accel_xy_angle_max data_store_memory; roll_target data_store_memory; pitch_target data_store_memory; POSCONTROL_ACCEL_XY_MAX data_store_memory; recalc_leash_xy data_store_memory; POSCONTROL_SPEED data_store_memory; reset_desired_vel_to_pos data_store_memory; POSCONTROL_OVERSPEED_GAIN_Z data_store_memory; POSCONTROL_JERK_RATIO data_store_memory; accel_last_z_cms data_store_memory; is_active_z data_store_memory; POSCONTROL_STOPPING_DIST_DOWN_MAX data_store_memory; POSCONTROL_STOPPING_DIST_UP_MAX data_store_memory; is_active_xy data_store_memory; attitude_target_quat data_store_memory; attitude_target_ang_vel data_store_memory; thrust_error_angle data_store_memory; rate_target_ang_vel data_store_memory; gyro_z data_store_memory; ang_vel_roll_max data_store_memory; ang_vel_pitch_max data_store_memory; ang_vel_yaw_max data_store_memory; AC_ATTITUDE_THRUST_ERROR_ANGLE data_store_memory; rate_bf_ff_enabled data_store_memory; attitude_ang_error data_store_memory; p_angle_yaw data_store_memory; AC_ATTITUDE_ACCEL_Y_CONTROLLER_MAX_RADSS data_store_memory; use_sqrt_controller data_store_memory; p_angle_roll data_store_memory; AC_ATTITUDE_ACCEL_RP_CONTROLLER_MIN_RADSS data_store_memory; AC_ATTITUDE_ACCEL_RP_CONTROLLER_MAX_RADSS data_store_memory; p_angle_pitch data_store_memory; accel_pitch_max data_store_memory; accel_yaw_max data_store_memory; accel_roll_max data_store_memory; AC_ATTITUDE_ACCEL_Y_CONTROLLER_MIN_RADSS data_store_memory; attitude_target_euler_angle data_store_memory; input_tc data_store_memory; attitude_target_euler_rate data_store_memory; slew_yaw data_store_memory; rate_pitch_pid_reset_filter data_store_memory; rate_pitch_pid_input data_store_memory; rate_pitch_pid_derivative data_store_memory; rate_pitch_pid_integrator data_store_memory; motors_limit_roll_pitch data_store_memory; ATC_RAT_PIT_D data_store_memory; ATC_RAT_PIT_FF data_store_memory; ATC_RAT_PIT_FILT data_store_memory; ATC_RAT_PIT_I data_store_memory; ATC_RAT_PIT_IMAX data_store_memory; ATC_RAT_PIT_P data_store_memory; ATC_RAT_RLL_D data_store_memory; ATC_RAT_RLL_FF data_store_memory; ATC_RAT_RLL_FILT data_store_memory; ATC_RAT_RLL_I data_store_memory; ATC_RAT_RLL_IMAX data_store_memory; ATC_RAT_RLL_P data_store_memory; rate_roll_pid_reset_filter data_store_memory; rate_roll_pid_input data_store_memory; rate_roll_pid_derivative data_store_memory; rate_roll_pid_integrator data_store_memory; ATC_RAT_YAW_D data_store_memory; ATC_RAT_YAW_FF data_store_memory; ATC_RAT_YAW_FILT data_store_memory; ATC_RAT_YAW_I data_store_memory; ATC_RAT_YAW_IMAX data_store_memory; ATC_RAT_YAW_P data_store_memory; rate_yaw_pid_reset_filter data_store_memory; rate_yaw_pid_input data_store_memory; rate_yaw_pid_derivative data_store_memory; rate_yaw_pid_integrator data_store_memory; motors_limit_yaw data_store_memory; gyro_x data_store_memory; gyro_y data_store_memory; inint data_store_memory; AP_MOTORS_MATRIX_YAW_FACTOR_CCW data_store_memory; AP_MOTORS_MATRIX_YAW_FACTOR_CW data_store_memory; pitch_factor data_store_memory; roll_factor data_store_memory; yaw_factor data_store_memory; throttle_in data_store_memory; throttle_cutoff_frequency data_store_memory; POSCONTROL_THROTTLE_CUTOFF_FREQ data_store_memory; throttle_filter data_store_memory; armed data_store_memory; roll_in data_store_memory; pitch_in data_store_memory; yaw_in data_store_memory; thrust_boost_ratio data_store_memory; thrust_rpyt_out data_store_memory; limit_roll_pitch data_store_memory; yaw_headroom data_store_memory; thrust_boost data_store_memory; limit_yaw data_store_memory; current_tilt data_store_memory; air_density_ratio data_store_memory; thrust_slew_time data_store_memory; attitude_error_vector data_store_memory; Kx data_store_memory; target_yaw_rate data_store_memory; climb_rate_cms data_store_memory; mode data_store_memory; mode_L1 data_store_memory; hgt_dem_cm data_store_memory; EAS_dem_cm data_store_memory; arspeed_filt data_store_memory; arspeed_temp data_store_memory; loc_origin data_store_memory; roll_target_pilot data_store_memory; pitch_target_pilot data_store_memory; center_WP data_store_memory; radius data_store_memory; loiter_direction data_store_memory; prev_WP data_store_memory; next_WP data_store_memory; dist_min data_store_memory; loc data_store_memory; tail_tilt data_store_memory; p_tail_tilt data_store_memory; p_tilt_pitch_target data_store_memory; disable_integrator_pitch data_store_memory; disable_integrator_roll data_store_memory; disable_integrator_yaw data_store_memory; aspeed_c2p data_store_memory; p_plane_c2p data_store_memory; yaw_max_c2p data_store_memory; weathervane_min_roll data_store_memory; weathervane_gain data_store_memory; yaw_rate_max data_store_memory; weathervane_last_output data_store_memory; POSCONTROL_ACC_Z_FILT_HZ_c2p data_store_memory; inint_hgt data_store_memory; desired_rate_roll data_store_memory; desired_rate_pitch data_store_memory; PathModeOut_sl data_store_memory; tail_tilt_p2c data_store_memory; tail_tilt_c2p data_store_memory; tail_tilt_rate data_store_memory; aspeed_c2ps data_store_memory; roll_ff_pitch_inint data_store_memory; K_FF_yaw_inint data_store_memory; POSCONTROL_ACC_Z_FILT_HZ_inint data_store_memory; POSCONTROL_ACC_Z_I_inint data_store_memory; POSCONTROL_VEL_XY_I_inint data_store_memory; ATC_RAT_PIT_I_inint data_store_memory; ATC_RAT_RLL_I_inint data_store_memory; ATC_RAT_YAW_I_inint data_store_memory; p_ff_throttle data_store_memory; vel_forward_last_pct data_store_memory; vel_forward_gain data_store_memory; vel_forward_min_pitch data_store_memory; vel_forward_tail_tilt_max data_store_memory; aspeed_cp data_store_memory; p_plane_cp data_store_memory; thr_out_min data_store_memory; pitch_target_p2c data_store_memory; k_throttle_c2p data_store_memory; throttle_off_rate data_store_memory; ff_throttle data_store_memory; throttle_ground data_store_memory; plane_mode data_store_memory; pwm_tail data_store_memory; yaw_in_max data_store_memory; pitch_target_c2p data_store_memory; take_off_land data_store_memory; vel_forward_integrator data_store_memory; algo_remote_ct_st data_store_memory; algo_dbg_param data_store_memory; Curr_sate data_store_memory; L1_radius data_store_memory; k_aileronL data_store_memory; k_aileronR data_store_memory; k_alieron_o output; k_elevator_o output; k_rudder_o output; k_aileronL_o output; k_aileronR_o output; tail_tilt_o output; pwm_out_o output; p_plane_p2c data_store_memory; pwm_tail_o output; POSCONTROL_THROTTLE_CUTOFF_FREQ_p2c data_store_memory; Fix2Rotor_delay_s data_store_memory; p_k_elevator_c2p data_store_memory; POSCONTROL_THROTTLE_CUTOFF_FREQ_inint data_store_memory; gains_D_pitch_inint data_store_memory; gains_D_roll_inint data_store_memory; thr_out_min_inint data_store_memory; spdWeight_inint data_store_memory; thr_out_min_c2p data_store_memory; heading_hold data_store_memory; k_flap_o output; k_flap data_store_memory; k_flap_TakeOff data_store_memory; k_flap_Land data_store_memory
function [k_alieron_o,k_elevator_o,k_rudder_o,k_aileronL_o,k_aileronR_o,tail_tilt_o,pwm_out_o,pwm_tail_o,k_flap_o] =copter_plane_run
global plane_mode
global k_aileron
global k_elevator
global k_rudder
global k_aileronL
global k_aileronR
global tail_tilt
global pwm_out
global pwm_tail
global k_flap
%     switch plane_mode
%         case ENUM_plane_mode.V1000
%             run_V1000();
%         case ENUM_plane_mode.V10
%             run_V10();
%         case ENUM_plane_mode.V10s
%             run_V10s();
%         otherwise
%             run_V10();
%     end 
% run_remote();
% load_Curr_sate();
% loc_run();
load_inint();

    switch plane_mode
        case ENUM_plane_mode.V1000
            run_V1000();
        case ENUM_plane_mode.V10
            run_V10();
        case ENUM_plane_mode.V10s
            run_V10s();
        otherwise
            run_V10();
    end 
run_servo_pwm_adj();
k_alieron_o= k_aileron;
k_elevator_o= k_elevator;
k_rudder_o= k_rudder;
k_aileronL_o= k_aileronL;
k_aileronR_o= k_aileronR;
tail_tilt_o= tail_tilt;
pwm_out_o= pwm_out;
pwm_tail_o= pwm_tail;
k_flap_o=k_flap;
end
